simulink model "SySControlPMSM"  (R2022a)
settings: Solver=VariableStepAuto  StartTime=0.0  StopTime=10.0  RelTol=1e-3
values from neighbouring files (symbols this model uses):
  Ts = 2e-06    [matlab.mat]
undefined symbols (not defined in the file or in its folder): DiscIntNeverNeededParam, Ion, Lithium
libraries: spsSeriesRLCBranchLib x2, spsVoltageMeasurementLib x2, spsParallelRLCBranchLib x1, spsMutualInductanceLib x1, spsUniversalBridgeLib x1, spsCurrentMeasurementLib x1, spsBatteryLib x1, spsPWMGenerator2LevelLib x1, spsPermanentMagnetSynchronousMachineLib x1, spspowerguiLib x1
settings Model: Creator=crow  LastModifiedBy=crow

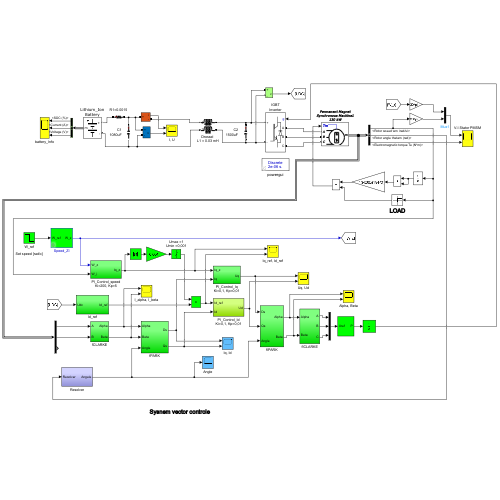
[thumbnail: Simulink's stored preview of the top-level diagram]
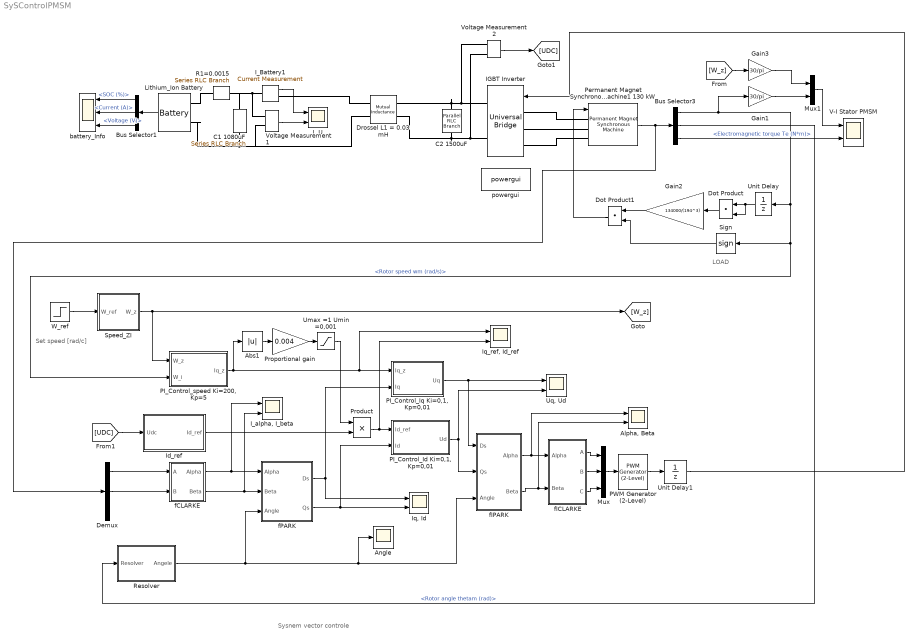
== system SySControlPMSM ==
  note: LOAD
  note: Sysnem vector controle
  note: Set speed [rad/c]
  Abs1 : Abs  SaturateOnIntegerOverflow=off
  "Alpha, Beta" : Scope  NumInputPorts=2
  Angle : Scope
  Bus Selector1 : BusSelector  OutputSignals=SOC (%),Current (A),Voltage (V)
  Bus Selector3 : BusSelector  OutputSignals=Rotor speed wm (rad/s),Rotor angle thetam (rad),Electromagnetic torque Te (N*m)
  "C1 1080uF " : spsSeriesRLCBranchLib/Series RLC Branch  LConnTagsString=__new0  RConnTagsString=__new0  BranchType=C  Resistance=0.0001  Inductance=1e-3  SetiL0=off  InitialCurrent=0  Capacitance=1080e-6  Setx0=on  InitialVoltage=700  Measurements=None
  C2 1500uF : spsParallelRLCBranchLib/Parallel RLC Branch  LConnTagsString=a  RConnTagsString=__new0  BranchType=C  Resistance=10000  Inductance=inf  SetiL0=off  InitialCurrent=0  Capacitance=1500e-6  Setx0=on  InitialVoltage=800  Measurements=None
  Demux : Demux  Outputs=3
  Dot Product : DotProduct  OutDataTypeStr=Inherit: Inherit via internal rule
  Dot Product1 : DotProduct  OutDataTypeStr=Inherit: Inherit via internal rule
  Drossel L1 = 0.03 mH : spsMutualInductanceLib/Mutual Inductance  LConnTagsString=a|b  RConnTagsString=A|B  TypeOfMutual=Two or three windings with equal mutual terms  NumberOfWindings=3  SelfImpedance1=[0.002 0.03e-03]  SelfImpedance2=[ 0.002 0.03e-03]  ThreeWindings=off  SelfImpedance3=[ 1.1 1.1e-03]  MutualImpedance=[0.0019 0.029e-03]  InductanceMatrix="[1.0 0.9  0.9 ;  0.9 1.0  0.9;  0.9 0.9 1.0 ] * 1e-3"  ResistanceMatrix="[1.0 0.9  0.9 ;  0.9 1.0  0.9;  0.9 0.9 1.0 ]"  Measurements=None
      settings: SourceProductBaseCode=PS
  Gain1 : Gain  Gain=30/pi  SaturateOnIntegerOverflow=on  OutDataTypeStr=Inherit: Same as input  ParamDataTypeStr=Inherit: Same as input
  Gain2 : Gain  Gain=134000/(194^3)  SaturateOnIntegerOverflow=on  OutDataTypeStr=Inherit: Same as input  ParamDataTypeStr=Inherit: Same as input
  Gain3 : Gain  Gain=30/pi  SaturateOnIntegerOverflow=on  OutDataTypeStr=Inherit: Same as input  ParamDataTypeStr=Inherit: Same as input
  "I, U" : Scope  NumInputPorts=2
  IGBT Inverter : spsUniversalBridgeLib/Universal Bridge  Arms=3  SnubberResistance=1e5  SnubberCapacitance=inf  Device=IGBT / Diodes  Ron=0.1e-3  Lon=0  ForwardVoltages="[  0  0  ]"  ForwardVoltage=0  GTOparameters=[ 10e-6 , 20e-6 ]  IGBTparameters=[ 1e-6 , 2e-6 ]  Measurements=Device currents  Measurements_2=None  converterType=Rectifier
  I_Battery1 : spsCurrentMeasurementLib/Current Measurement  PhasorSimulation=off  OutputType=Complex  PSBequivalent=0
  "I_alpha, I_beta" : Scope  NumInputPorts=2
  Id_ref : Subsystem
  "Iq, Id" : Scope  NumInputPorts=2
  "Iq_ref, Id_ref" : Scope  NumInputPorts=2
  Lithium_Ion Battery : spsBatteryLib/Battery  BatType=Lithium-Ion  ShowTempParam=off  ThermalPreset=no  ShowAgeParam=off  NomV=600  NomQ=710  SOC=5  Batt_Tr=300  PresetModel=off  MaxQ=710  MinV=550  FullV=700  Dis_rate=308.6957  R=0.0092958  Normal_OP=642.087  expZone="[650.0547      34.88261]"  current=[6.5 13 32.5]  Units=Time  Tci=20  NomT=25  T2=0  MaxQ2=2.208  FullV2=3.45  Normal_OP2=2.8  expZone2="[3.22        0.23]"  Rca=0.6  ti=1000  Dp=0  Neq0=0  Tsim=1e6  Ta1=25  Qeol=5.4*0.9  Reol=0.013333*1.2  Char_age=[2.3478, 3]  Dis_age=[2.3478, 10]  N1=1500  N2=10500  N3=1000  N4=1400  Ta2=45  N5=950
  Mux : Mux  Inputs=3
  Mux1 : Mux  Inputs=2
  "PI_Control_Id Ki=0,1, Kp=0,01" : Subsystem
  "PI_Control_Iq Ki=0,1, Kp=0,01" : Subsystem
  "PI_Control_speed Ki=200, Kp=5" : Subsystem
  PWM Generator (2-Level) : spsPWMGenerator2LevelLib/PWM Generator (2-Level)  ModulatorType=Three-phase bridge (6 pulses)  ModulatorMode=Unsynchronized  Fc=6000  Pc=0  nF=27  MinMax="[ -1  1 ]"  SamplingTechnique=Natural  ModulatingSignals=off  m=0.8  Freq=60  Phase=0  Ts=Ts  ShowCarrierOutport=off
  Permanent Magnet Synchronous Machine1 130 kW : spsPermanentMagnetSynchronousMachineLib/Permanent Magnet Synchronous Machine  NbPhases=3  FluxDistribution=Sinusoidal  RotorType=Salient-pole  MechanicalLoad=Torque Tm  PresetModel=No  ShowDetailedParameters=on  MeasurementBus=off  Resistance=0.01  Inductance=8.5e-3  dqInductances=[0.3466e-3,0.71918e-3]  La=0.00153  MachineConstant=Torque Constant (N.m / A_peak)  Flux=0.178  VoltageCst=161.4281  TorqueCst=1.335  Flat=120  Mechanical=[ 0.22,0,5]  PolePairs=4  InitialConditions=[0,0, 0,0]  InitialConditions5ph=[0 0 0 0 0 0]  RefAngle=90 degrees behind phase A axis (modified Park)  IterativeDiscreteModel=Trapezoidal non iterative  TsBlock=-1  TsPowergui=0
  Product : Product
  Proportional gain : Gain  Gain=0.004  SaturateOnIntegerOverflow=on  OutDataTypeStr=Inherit: Same as input  ParamDataTypeStr=Inherit: Same as input
  R1=0.0015 : spsSeriesRLCBranchLib/Series RLC Branch  LConnTagsString=__new0  RConnTagsString=__new0  BranchType=R  Resistance=0.001  Inductance=1e-3  SetiL0=off  InitialCurrent=0  Capacitance=1e-6  Setx0=off  InitialVoltage=0  Measurements=None
  Resolver : Subsystem
  Sign : Signum
  Speed_ZI : Subsystem  mask{TR=2, TT=2}
      mask prompts: TR "Время разгона c."; TT "Время торможения с."
  Umax =1 Umin =0,001 : Saturate  UpperLimit=1  LowerLimit=0.001
  Unit Delay : UnitDelay  SampleTime=Ts  HasFrameUpgradeWarning=on
  Unit Delay1 : UnitDelay  SampleTime=Ts  HasFrameUpgradeWarning=on
  "Uq, Ud" : Scope  NumInputPorts=2
  V-I Stator PMSM : Scope  NumInputPorts=2
  Voltage Measurement1 : spsVoltageMeasurementLib/Voltage Measurement  PhasorSimulation=off  OutputType=Complex  PSBequivalent=0
  Voltage Measurement2 : spsVoltageMeasurementLib/Voltage Measurement  PhasorSimulation=off  OutputType=Complex  PSBequivalent=0
  W_ref : Step  Time=3  Before=100  After=-194  SampleTime=Ts
  battery_Info : Scope  NumInputPorts=3
  fCLARKE : Subsystem
  fICLARKE : Subsystem
  fIPARK : Subsystem
  fPARK : Subsystem
  powergui : spspowerguiLib/powergui  SimulationMode=Discrete  SampleTime=Ts  frequency=60  Iterations=50  frequencyindice=0  Pbase=100e6  ErrMax=1e-4  UnitsV=kV  UnitsW=MW  buscounter=0  FunctionMessages=off  echomessages=off  EnableUseOfTLC=off  CurrentSourceSwitches=off  DisableSnubberDevices=off  DisableRonSwitches=off  DisableVfSwitches=off  DisplayEquations=off  AutomaticDiscreteSolvers=off  SolverType=Tustin  Interpol=off  ExternalGateDelay=off  methode=off  Ts=0  x0status=blocks  SPID=on  SwTol=0  HookPort=off  NonlinearTolerance=1e-4  nMaxIteration=100  ContinueOnMaxIteration=off  RestoreLinks=warning  ResistiveCurrentMeasurement=off  Frange=[0:2:500]  Ylog=off  Xlog=on  ShowGrid=off  save=off  variable=ZData  structure=0  ZoomFFT=on  StartTime=0.0  cycles=1  DisplayStyle=1  fundamental=60  FreqAxis=off  MaxFrequency=1000  frequencyindicesteady=1  RmsSteady=1  display=off
  wires:
  Voltage Measurement1/1 -> "I, U"/2
  Bus Selector1/2 -> battery_Info/2  "<Current (A)>"
  Bus Selector1/1 -> battery_Info/1  "<SOC (%)>"
  Lithium_Ion Battery/1 -> Bus Selector1/1
  Bus Selector1/3 -> battery_Info/3  "<Voltage (V)>"
  I_Battery1/1 -> "I, U"/1
  Sign/1 -> Dot Product1/2
  Gain2/1 -> Dot Product1/1
  Bus Selector3/1 -> Gain1/1, Unit Delay/1, "PI_Control_speed Ki=200, Kp=5"/2(W_i), Sign/1  "<Rotor speed wm (rad/s)>"
  Unit Delay/1 -> Dot Product/2, Dot Product/1
  Dot Product/1 -> Gain2/1
  Dot Product1/1 -> Permanent Magnet Synchronous Machine1 130 kW/1
  Bus Selector3/3 -> V-I Stator PMSM/2  "<Electromagnetic torque Te (N*m)>"
  Mux1/1 -> V-I Stator PMSM/1
  Gain1/1 -> Mux1/2
  fCLARKE/2(Beta) -> "I_alpha, I_beta"/2, fPARK/2(Beta)
  Permanent Magnet Synchronous Machine1 130 kW/1 -> Demux/1, Bus Selector3/1
  Id_ref/1(Id_ref) -> Product/2
  "PI_Control_speed Ki=200, Kp=5"/1(Iq_z) -> Abs1/1, "Iq_ref, Id_ref"/1, "PI_Control_Iq Ki=0,1, Kp=0,01"/1(Iq_z)
  fCLARKE/1(Alpha) -> fPARK/1(Alpha), "I_alpha, I_beta"/1
  Abs1/1 -> Proportional gain/1
  fICLARKE/2(B) -> Mux/2
  "PI_Control_Id Ki=0,1, Kp=0,01"/1(Ud) -> fIPARK/2(Qs), "Uq, Ud"/2
  fPARK/1(Ds) -> "PI_Control_Iq Ki=0,1, Kp=0,01"/2(Iq), "Iq, Id"/1
  PWM Generator (2-Level)/1 -> Unit Delay1/1
  fICLARKE/1(A) -> Mux/1
  W_ref/1 -> Speed_ZI/1(W_ref)
  Mux/1 -> PWM Generator (2-Level)/1
  "PI_Control_Iq Ki=0,1, Kp=0,01"/1(Uq) -> "Uq, Ud"/1, fIPARK/1(Ds)
  fICLARKE/3(C) -> Mux/3
  fPARK/2(Qs) -> "PI_Control_Id Ki=0,1, Kp=0,01"/2(Id), "Iq, Id"/2
  Umax =1 Umin =0,001/1 -> Product/1
  [UDC] -> Id_ref/1(Udc)
  Demux/1 -> fCLARKE/1(A)
  fIPARK/2(Beta) -> "Alpha, Beta"/2, fICLARKE/2(Beta)
  Proportional gain/1 -> Umax =1 Umin =0,001/1
  Resolver/1(Angele) -> fPARK/3(Angle), Angle/1, fIPARK/3(Angle)
  fIPARK/1(Alpha) -> "Alpha, Beta"/1, fICLARKE/1(Alpha)
  Speed_ZI/1(W_z) -> [W_z], "PI_Control_speed Ki=200, Kp=5"/1(W_z)
  Demux/2 -> fCLARKE/2(B)
  Product/1 -> "Iq_ref, Id_ref"/2, "PI_Control_Id Ki=0,1, Kp=0,01"/1(Id_ref)
  Unit Delay1/1 -> IGBT Inverter/1
  Gain3/1 -> Mux1/1
  [W_z] -> Gain3/1
  Bus Selector3/2 -> Resolver/1(Resolver)  "<Rotor angle thetam (rad)>"
  Voltage Measurement2/1 -> [UDC]
  connections:
  IGBT Inverter/LConn1 -- Permanent Magnet Synchronous Machine1 130 kW/LConn1
  IGBT Inverter/LConn2 -- Permanent Magnet Synchronous Machine1 130 kW/LConn2
  IGBT Inverter/LConn3 -- Permanent Magnet Synchronous Machine1 130 kW/LConn3
  C2 1500uF/LConn1 -- Drossel L1 = 0.03 mH/RConn1 -- Voltage Measurement2/LConn1 -- IGBT Inverter/RConn1
  C2 1500uF/RConn1 -- Drossel L1 = 0.03 mH/RConn2 -- Voltage Measurement2/LConn2 -- IGBT Inverter/RConn2
  "C1 1080uF "/RConn1 -- Drossel L1 = 0.03 mH/LConn2 -- Voltage Measurement1/LConn2 -- Lithium_Ion Battery/LConn2
  I_Battery1/LConn1 -- "C1 1080uF "/LConn1 -- R1=0.0015/RConn1 -- Voltage Measurement1/LConn1
  R1=0.0015/LConn1 -- Lithium_Ion Battery/LConn1
  Drossel L1 = 0.03 mH/LConn1 -- I_Battery1/RConn1

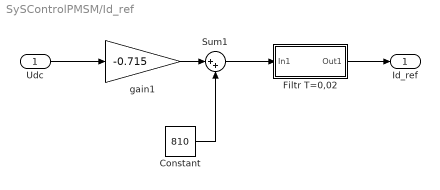
== system SySControlPMSM/Id_ref ==
  Udc : Inport
  " gain1" : Gain  Gain=-0.715  SaturateOnIntegerOverflow=on  OutDataTypeStr=Inherit: Same as input  ParamDataTypeStr=Inherit: Same as input
  Constant : Constant  Value=810
  Filtr T=0,02 : Subsystem
  Sum1 : Sum  Inputs=|++  InputSameDT=on  SaturateOnIntegerOverflow=on  OutDataTypeStr=Inherit: Same as first input
  Id_ref : Outport
  wires:
  Constant/1 -> Sum1/2
  " gain1"/1 -> Sum1/1
  Udc/1 -> " gain1"/1
  Sum1/1 -> Filtr T=0,02/1(In1)
  Filtr T=0,02/1(Out1) -> Id_ref/1

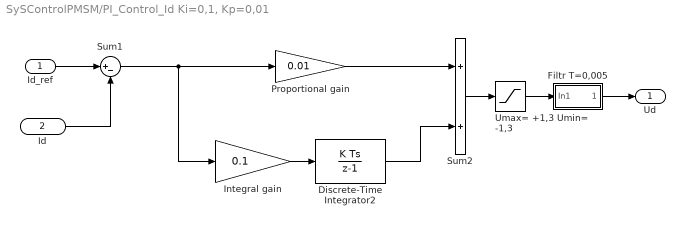
== system SySControlPMSM/PI_Control_Id Ki=0,1, Kp=0,01 ==
  Id_ref : Inport
  Id : Inport  Port=2
  Discrete-Time Integrator2 : DiscreteIntegrator  SampleTime=-1  UpperSaturationLimit=3  LowerSaturationLimit=-3  ICPrevOutput=DiscIntNeverNeededParam  ICPrevScaledInput=DiscIntNeverNeededParam
  Filtr T=0,005 : Subsystem
  Integral gain : Gain  Gain=0.1  SaturateOnIntegerOverflow=on  OutDataTypeStr=Inherit: Same as input  ParamDataTypeStr=Inherit: Same as input
  Proportional gain : Gain  Gain=0.01  SaturateOnIntegerOverflow=on  OutDataTypeStr=Inherit: Same as input  ParamDataTypeStr=Inherit: Same as input
  Sum1 : Sum  Inputs=|+-  InputSameDT=on  SaturateOnIntegerOverflow=on  OutDataTypeStr=Inherit: Same as first input
  Sum2 : Sum  InputSameDT=on  SaturateOnIntegerOverflow=on  OutDataTypeStr=Inherit: Same as first input
  Umax= +1,3 Umin= -1,3 : Saturate  UpperLimit=1.3  LowerLimit=-1.3
  Ud : Outport
  wires:
  Integral gain/1 -> Discrete-Time Integrator2/1
  Sum2/1 -> Umax= +1,3 Umin= -1,3/1
  Id_ref/1 -> Sum1/1
  Id/1 -> Sum1/2
  Discrete-Time Integrator2/1 -> Sum2/2
  Proportional gain/1 -> Sum2/1
  Umax= +1,3 Umin= -1,3/1 -> Filtr T=0,005/1(In1)
  Sum1/1 -> Integral gain/1, Proportional gain/1
  Filtr T=0,005/1(Out1) -> Ud/1

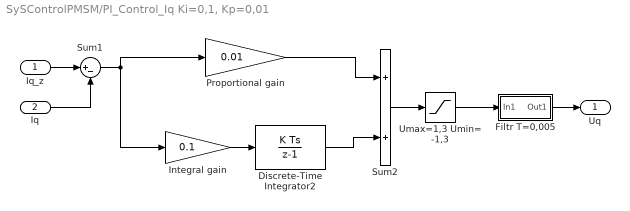
== system SySControlPMSM/PI_Control_Iq Ki=0,1, Kp=0,01 ==
  Iq_z : Inport
  Iq : Inport  Port=2
  Discrete-Time Integrator2 : DiscreteIntegrator  SampleTime=-1  UpperSaturationLimit=100  LowerSaturationLimit=-100  ICPrevOutput=DiscIntNeverNeededParam  ICPrevScaledInput=DiscIntNeverNeededParam
  Filtr T=0,005 : Subsystem
  Integral gain : Gain  Gain=0.1  SaturateOnIntegerOverflow=on  OutDataTypeStr=Inherit: Same as input  ParamDataTypeStr=Inherit: Same as input
  Proportional gain : Gain  Gain=0.01  SaturateOnIntegerOverflow=on  OutDataTypeStr=Inherit: Same as input  ParamDataTypeStr=Inherit: Same as input
  Sum1 : Sum  Inputs=|+-  InputSameDT=on  SaturateOnIntegerOverflow=on  OutDataTypeStr=Inherit: Same as first input
  Sum2 : Sum  InputSameDT=on  SaturateOnIntegerOverflow=on  OutDataTypeStr=Inherit: Same as first input
  Umax=1,3 Umin= -1,3 : Saturate  UpperLimit=1.3  LowerLimit=-1.3
  Uq : Outport
  wires:
  Iq/1 -> Sum1/2
  Iq_z/1 -> Sum1/1
  Sum2/1 -> Umax=1,3 Umin= -1,3/1
  Integral gain/1 -> Discrete-Time Integrator2/1
  Proportional gain/1 -> Sum2/1
  Discrete-Time Integrator2/1 -> Sum2/2
  Umax=1,3 Umin= -1,3/1 -> Filtr T=0,005/1(In1)
  Sum1/1 -> Integral gain/1, Proportional gain/1
  Filtr T=0,005/1(Out1) -> Uq/1

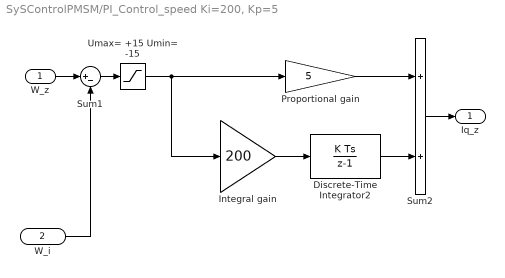
== system SySControlPMSM/PI_Control_speed Ki=200, Kp=5 ==
  W_z : Inport
  W_i : Inport  Port=2
  Discrete-Time Integrator2 : DiscreteIntegrator  SampleTime=Ts  UpperSaturationLimit=500  LowerSaturationLimit=-500  ICPrevOutput=DiscIntNeverNeededParam  ICPrevScaledInput=DiscIntNeverNeededParam
  Integral gain : Gain  Gain=200  SaturateOnIntegerOverflow=on  OutDataTypeStr=Inherit: Same as input  ParamDataTypeStr=Inherit: Same as input
  Proportional gain : Gain  Gain=5  SaturateOnIntegerOverflow=on  OutDataTypeStr=Inherit: Same as input  ParamDataTypeStr=Inherit: Same as input
  Sum1 : Sum  Inputs=|+-  InputSameDT=on  SaturateOnIntegerOverflow=on  OutDataTypeStr=Inherit: Same as first input
  Sum2 : Sum  InputSameDT=on  SaturateOnIntegerOverflow=on  OutDataTypeStr=Inherit: Same as first input
  Umax= +15 Umin= -15 : Saturate  UpperLimit=15  LowerLimit=-15
  Iq_z : Outport
  wires:
  Integral gain/1 -> Discrete-Time Integrator2/1
  Sum2/1 -> Iq_z/1
  W_i/1 -> Sum1/2
  Proportional gain/1 -> Sum2/1
  Discrete-Time Integrator2/1 -> Sum2/2
  Sum1/1 -> Umax= +15 Umin= -15/1
  W_z/1 -> Sum1/1
  Umax= +15 Umin= -15/1 -> Integral gain/1, Proportional gain/1

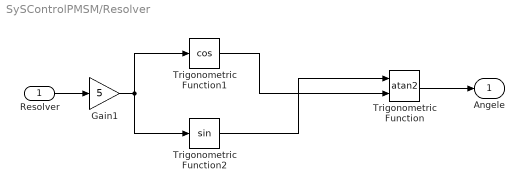
== system SySControlPMSM/Resolver ==
  Resolver : Inport
  Gain1 : Gain  Gain=5  SaturateOnIntegerOverflow=on  OutDataTypeStr=Inherit: Same as input  ParamDataTypeStr=Inherit: Same as input
  Trigonometric Function : Trigonometry  Operator=atan2
  Trigonometric Function1 : Trigonometry  Operator=cos
  Trigonometric Function2 : Trigonometry
  Angele : Outport
  wires:
  Resolver/1 -> Gain1/1
  Gain1/1 -> Trigonometric Function1/1, Trigonometric Function2/1
  Trigonometric Function2/1 -> Trigonometric Function/1
  Trigonometric Function1/1 -> Trigonometric Function/2
  Trigonometric Function/1 -> Angele/1

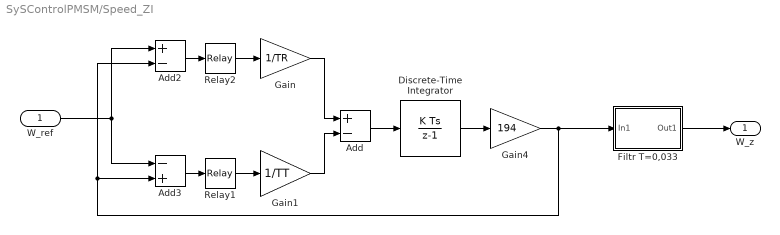
== system SySControlPMSM/Speed_ZI ==
  W_ref : Inport
  Add : Sum  Inputs=+-
  Add2 : Sum  Inputs=+-
  Add3 : Sum  Inputs=-+
  Discrete-Time Integrator : DiscreteIntegrator  SampleTime=Ts  ICPrevOutput=DiscIntNeverNeededParam  ICPrevScaledInput=DiscIntNeverNeededParam
  Filtr T=0,033 : Subsystem
  Gain : Gain  Gain=1/TR
  Gain1 : Gain  Gain=1/TT
  Gain4 : Gain  Gain=194
  Relay1 : Relay  OnSwitchValue=-0.001  OffSwitchValue=-0.002
  Relay2 : Relay  OnSwitchValue=0.001  OffSwitchValue=0
  W_z : Outport
  wires:
  Relay2/1 -> Gain/1
  Gain/1 -> Add/1
  Relay1/1 -> Gain1/1
  Gain1/1 -> Add/2
  Add2/1 -> Relay2/1
  Add3/1 -> Relay1/1
  Discrete-Time Integrator/1 -> Gain4/1
  Add/1 -> Discrete-Time Integrator/1
  W_ref/1 -> Add2/1, Add3/1
  Gain4/1 -> Filtr T=0,033/1(In1), Add3/2, Add2/2
  Filtr T=0,033/1(Out1) -> W_z/1

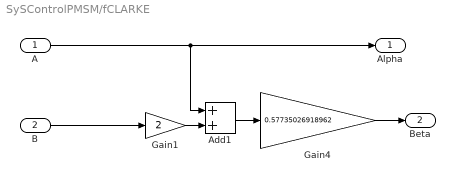
== system SySControlPMSM/fCLARKE ==
  A : Inport
  B : Inport  Port=2
  Add1 : Sum
  Gain1 : Gain  Gain=2
  Gain4 : Gain  Gain=0.57735026918962
  Alpha : Outport
  Beta : Outport  Port=2
  wires:
  Gain4/1 -> Beta/1
  Gain1/1 -> Add1/2
  Add1/1 -> Gain4/1
  B/1 -> Gain1/1
  A/1 -> Add1/1, Alpha/1

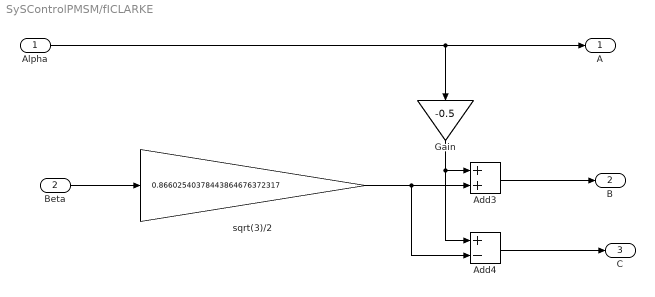
== system SySControlPMSM/fICLARKE ==
  Alpha : Inport
  Beta : Inport  Port=2
  Add3 : Sum
  Add4 : Sum  Inputs=+-
  Gain : Gain  Gain=-0.5
  sqrt(3)/2 : Gain  Gain=0.86602540378443864676372317
  A : Outport
  B : Outport  Port=2
  C : Outport  Port=3
  wires:
  Beta/1 -> sqrt(3)/2/1
  Alpha/1 -> A/1, Gain/1
  sqrt(3)/2/1 -> Add4/2, Add3/2
  Gain/1 -> Add4/1, Add3/1
  Add3/1 -> B/1
  Add4/1 -> C/1

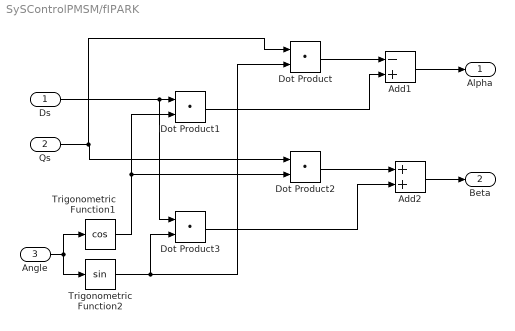
== system SySControlPMSM/fIPARK ==
  Ds : Inport
  Qs : Inport  Port=2
  Angle : Inport  Port=3
  Add1 : Sum  Inputs=-+
  Add2 : Sum
  Dot Product{,1..3} (4 alike) : DotProduct  OutDataTypeStr=Inherit: Inherit via internal rule
  Trigonometric Function1 : Trigonometry  Operator=cos
  Trigonometric Function2 : Trigonometry
  Alpha : Outport
  Beta : Outport  Port=2
  wires:
  Dot Product3/1 -> Add2/2
  Dot Product2/1 -> Add2/1
  Dot Product1/1 -> Add1/2
  Dot Product/1 -> Add1/1
  Add1/1 -> Alpha/1
  Add2/1 -> Beta/1
  Trigonometric Function1/1 -> Dot Product2/2, Dot Product1/2
  Trigonometric Function2/1 -> Dot Product/2, Dot Product3/2
  Angle/1 -> Trigonometric Function2/1, Trigonometric Function1/1
  Ds/1 -> Dot Product3/1, Dot Product1/1
  Qs/1 -> Dot Product/1, Dot Product2/1

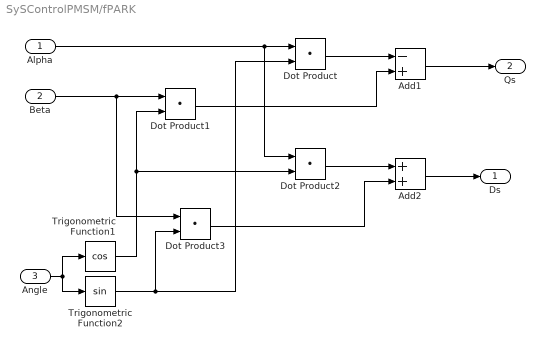
== system SySControlPMSM/fPARK ==
  Alpha : Inport
  Beta : Inport  Port=2
  Angle : Inport  Port=3
  Add1 : Sum  Inputs=-+
  Add2 : Sum
  Dot Product{,1..3} (4 alike) : DotProduct  OutDataTypeStr=Inherit: Inherit via internal rule
  Trigonometric Function1 : Trigonometry  Operator=cos
  Trigonometric Function2 : Trigonometry
  Ds : Outport
  Qs : Outport  Port=2
  wires:
  Dot Product/1 -> Add1/1
  Dot Product1/1 -> Add1/2
  Alpha/1 -> Dot Product2/1, Dot Product/1
  Beta/1 -> Dot Product3/1, Dot Product1/1
  Dot Product2/1 -> Add2/1
  Dot Product3/1 -> Add2/2
  Trigonometric Function2/1 -> Dot Product3/2, Dot Product/2
  Trigonometric Function1/1 -> Dot Product1/2, Dot Product2/2
  Angle/1 -> Trigonometric Function2/1, Trigonometric Function1/1
  Add1/1 -> Qs/1
  Add2/1 -> Ds/1

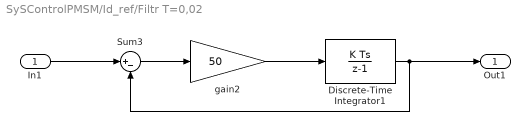
== system SySControlPMSM/Id_ref/Filtr T=0,02 ==
  In1 : Inport
  " gain2" : Gain  Gain=50  SaturateOnIntegerOverflow=on  OutDataTypeStr=Inherit: Same as input  ParamDataTypeStr=Inherit: Same as input
  Discrete-Time Integrator1 : DiscreteIntegrator  SampleTime=Ts  UpperSaturationLimit=3  LowerSaturationLimit=-3  ICPrevOutput=DiscIntNeverNeededParam  ICPrevScaledInput=DiscIntNeverNeededParam
  Sum3 : Sum  Inputs=|+-  InputSameDT=on  SaturateOnIntegerOverflow=on  OutDataTypeStr=Inherit: Same as first input
  Out1 : Outport
  wires:
  Sum3/1 -> " gain2"/1
  In1/1 -> Sum3/1
  Discrete-Time Integrator1/1 -> Out1/1, Sum3/2
  " gain2"/1 -> Discrete-Time Integrator1/1

== system SySControlPMSM/PI_Control_Id Ki=0,1, Kp=0,01/Filtr T=0,005 ==
  In1 : Inport
  Discrete-Time Integrator1 : DiscreteIntegrator  SampleTime=-1  UpperSaturationLimit=3  LowerSaturationLimit=-3  ICPrevOutput=DiscIntNeverNeededParam  ICPrevScaledInput=DiscIntNeverNeededParam
  Integral gain1 : Gain  Gain=200  SaturateOnIntegerOverflow=on  OutDataTypeStr=Inherit: Same as input  ParamDataTypeStr=Inherit: Same as input
  Sum3 : Sum  Inputs=|+-  InputSameDT=on  SaturateOnIntegerOverflow=on  OutDataTypeStr=Inherit: Same as first input
  Out1 : Outport
  wires:
  Discrete-Time Integrator1/1 -> Out1/1, Sum3/2
  Sum3/1 -> Integral gain1/1
  Integral gain1/1 -> Discrete-Time Integrator1/1
  In1/1 -> Sum3/1

== system SySControlPMSM/PI_Control_Iq Ki=0,1, Kp=0,01/Filtr T=0,005 ==
  In1 : Inport
  Discrete-Time Integrator1 : DiscreteIntegrator  SampleTime=-1  UpperSaturationLimit=3  LowerSaturationLimit=-3  ICPrevOutput=DiscIntNeverNeededParam  ICPrevScaledInput=DiscIntNeverNeededParam
  Integral gain1 : Gain  Gain=200  SaturateOnIntegerOverflow=on  OutDataTypeStr=Inherit: Same as input  ParamDataTypeStr=Inherit: Same as input
  Sum3 : Sum  Inputs=|+-  InputSameDT=on  SaturateOnIntegerOverflow=on  OutDataTypeStr=Inherit: Same as first input
  Out1 : Outport
  wires:
  In1/1 -> Sum3/1
  Integral gain1/1 -> Discrete-Time Integrator1/1
  Sum3/1 -> Integral gain1/1
  Discrete-Time Integrator1/1 -> Sum3/2, Out1/1

== system SySControlPMSM/Speed_ZI/Filtr T=0,033 ==
  In1 : Inport
  Add4 : Sum  Inputs=+-
  Discrete-Time Integrator1 : DiscreteIntegrator  SampleTime=Ts  ICPrevOutput=DiscIntNeverNeededParam  ICPrevScaledInput=DiscIntNeverNeededParam
  Gain2 : Gain  Gain=30
  Out1 : Outport
  wires:
  Discrete-Time Integrator1/1 -> Out1/1, Add4/2
  Add4/1 -> Gain2/1
  Gain2/1 -> Discrete-Time Integrator1/1
  In1/1 -> Add4/1
